simulink subsystem "convert_Info_to_angle"  (R2021a)
settings: Solver=VariableStepAuto  StartTime=0.0  StopTime=10.0  RelTol=1e-3
values from neighbouring files (symbols this model uses):
  init_time = 1.0    [common_data.sldd]
  ts_raspi = 0.005    [common_data.sldd]
settings Model: Creator=tshintai  LastModifiedBy=tshintai

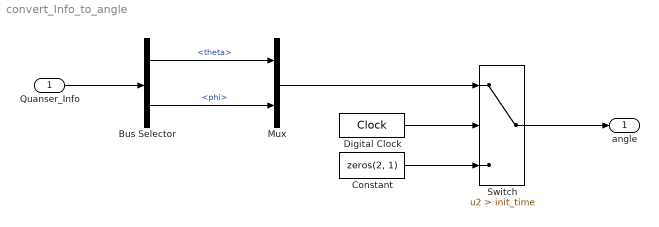
== system convert_Info_to_angle ==
  Quanser_Info : Inport
  Bus Selector : BusSelector  OutputSignals=theta,phi
  Constant : Constant  Value=zeros(2, 1)
  Digital Clock : DigitalClock  SampleTime=ts_raspi
  Mux : Mux  Inputs=2
  Switch : Switch  Criteria=u2 > Threshold  Threshold=init_time
  angle : Outport
  wires:
  Quanser_Info/1 -> Bus Selector/1
  Bus Selector/1 -> Mux/1  "<theta>"
  Bus Selector/2 -> Mux/2  "<phi>"
  Mux/1 -> Switch/1
  Digital Clock/1 -> Switch/2
  Switch/1 -> angle/1
  Constant/1 -> Switch/3
